simulink model "WholeBody"  (R2023b)
settings: Solver=daessc  StartTime=0.0  StopTime=10  RelTol=1e-3
undefined symbols (not defined in the file): Kd, Ki, Kp, LF, LFstates, LFtrqs, LR, LRstates, LRtrqs, RF, RFstates, RFtrqs, RR, RRstates, RRtrqs, X, Y, Z
libraries: sm_lib x57, nesl_utility x37, SignalEditorBlockLib x1
(part 3 of 3)

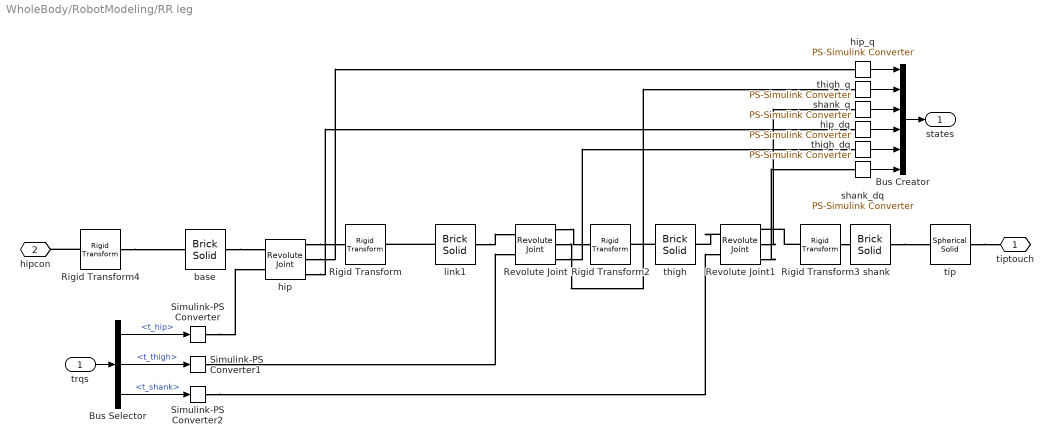
== system WholeBody/RobotModeling/RR leg ==
  trqs : Inport
  Bus Creator : BusCreator  Inputs=6
  Bus Selector : BusSelector  OutputSignals=t_hip,t_thigh,t_shank
  Revolute Joint : sm_lib/Joints/Revolute Joint  JointMode=Normal  SenseConstraintForce=off  SenseConstraintForceX=off  SenseConstraintForceY=off  SenseConstraintForceZ=off  SenseConstraintTorque=off  SenseConstraintTorqueX=off  SenseConstraintTorqueY=off  SenseConstraintTorqueZ=off  SenseTotalForce=off  SenseTotalForceX=off  SenseTotalForceY=off  SenseTotalForceZ=off  SenseTotalTorque=off  SenseTotalTorqueX=off  SenseTotalTorqueY=off  SenseTotalTorqueZ=off  CompositeWrenchDir=FollowerOnBase  CompositeWrenchFrame=BaseFrame  EquilibriumPosition=0  EquilibriumPositionUnits=deg  SpringStiffness=0  SpringStiffnessUnits=N*m/deg  DampingCoefficient=0  DampingCoefficientUnits=N*m/(deg/s)  TorqueActuationMode=InputTorque  MotionActuationMode=ComputedMotion  SensePosition=on  SenseVelocity=on  SenseAcceleration=off  SenseTorqueForce=off  SenseLowerLimitTorqueForce=off  SenseUpperLimitTorqueForce=off  LowerLimitSpecify=off  LowerLimitBound=-90  LowerLimitBoundUnits=deg  LowerLimitStiffness=1e4  LowerLimitStiffnessUnits=N*m/deg  LowerLimitDamping=10  LowerLimitDampingUnits=N*m/(deg/s)  LowerLimitTransitionRegionWidth=0.1  LowerLimitTransitionRegionWidthUnits=deg  UpperLimitSpecify=off  UpperLimitBound=90  UpperLimitBoundUnits=deg  UpperLimitStiffness=1e4  UpperLimitStiffnessUnits=N*m/deg  UpperLimitDamping=10  UpperLimitDampingUnits=N*m/(deg/s)  UpperLimitTransitionRegionWidth=0.1  UpperLimitTransitionRegionWidthUnits=deg  PositionTargetSpecify=off  PositionTargetPriority=High  PositionTargetValue=0  PositionTargetValueUnits=deg  VelocityTargetSpecify=off  VelocityTargetPriority=High  VelocityTargetValue=0  VelocityTargetValueUnits=deg/s
  Revolute Joint1 : sm_lib/Joints/Revolute Joint  JointMode=Normal  SenseConstraintForce=off  SenseConstraintForceX=off  SenseConstraintForceY=off  SenseConstraintForceZ=off  SenseConstraintTorque=off  SenseConstraintTorqueX=off  SenseConstraintTorqueY=off  SenseConstraintTorqueZ=off  SenseTotalForce=off  SenseTotalForceX=off  SenseTotalForceY=off  SenseTotalForceZ=off  SenseTotalTorque=off  SenseTotalTorqueX=off  SenseTotalTorqueY=off  SenseTotalTorqueZ=off  CompositeWrenchDir=FollowerOnBase  CompositeWrenchFrame=BaseFrame  EquilibriumPosition=0  EquilibriumPositionUnits=deg  SpringStiffness=0  SpringStiffnessUnits=N*m/deg  DampingCoefficient=0  DampingCoefficientUnits=N*m/(deg/s)  TorqueActuationMode=InputTorque  MotionActuationMode=ComputedMotion  SensePosition=on  SenseVelocity=on  SenseAcceleration=off  SenseTorqueForce=off  SenseLowerLimitTorqueForce=off  SenseUpperLimitTorqueForce=off  LowerLimitSpecify=off  LowerLimitBound=-90  LowerLimitBoundUnits=deg  LowerLimitStiffness=1e4  LowerLimitStiffnessUnits=N*m/deg  LowerLimitDamping=10  LowerLimitDampingUnits=N*m/(deg/s)  LowerLimitTransitionRegionWidth=0.1  LowerLimitTransitionRegionWidthUnits=deg  UpperLimitSpecify=off  UpperLimitBound=90  UpperLimitBoundUnits=deg  UpperLimitStiffness=1e4  UpperLimitStiffnessUnits=N*m/deg  UpperLimitDamping=10  UpperLimitDampingUnits=N*m/(deg/s)  UpperLimitTransitionRegionWidth=0.1  UpperLimitTransitionRegionWidthUnits=deg  PositionTargetSpecify=off  PositionTargetPriority=High  PositionTargetValue=20  PositionTargetValueUnits=deg  VelocityTargetSpecify=off  VelocityTargetPriority=High  VelocityTargetValue=0  VelocityTargetValueUnits=deg/s
  Rigid Transform : sm_lib/Frames and Transforms/Rigid Transform  TranslationMethod=Cartesian  TranslationStandardOffset=0  TranslationStandardOffsetUnits=m  TranslationStandardAxis=+Z  TranslationCartesianOffset=[0.1 0 0]  TranslationCartesianOffsetUnits=m  TranslationROffset=0  TranslationROffsetUnits=m  TranslationZOffset=0  TranslationZOffsetUnits=m  TranslationThetaOffset=0  TranslationThetaOffsetUnits=deg  RotationMethod=None  RotationAngleUnits=deg  RotationStandardAxis=+Z  RotationAngle=0.0  RotationArbitraryAxis=[0 0 1]  FollAlignAxisA=+X  BaseAlignAxisA=+Y  FollAlignAxisB=+Y  BaseAlignAxisB=+Z  RotationSequenceAxes=FollowerAxes  RotationSequence=XYX  RotationSequenceAngles=[0 0 0]  RotationSequenceAnglesUnits=deg  RotationMatrix=[1 0 0; 0 1 0; 0 0 1]  Quaternion=[1 0 0 0]
  Rigid Transform2 : sm_lib/Frames and Transforms/Rigid Transform  TranslationMethod=Cartesian  TranslationStandardOffset=0  TranslationStandardOffsetUnits=m  TranslationStandardAxis=+Z  TranslationCartesianOffset=[0 -0.4 0]  TranslationCartesianOffsetUnits=m  TranslationROffset=0  TranslationROffsetUnits=m  TranslationZOffset=0  TranslationZOffsetUnits=m  TranslationThetaOffset=0  TranslationThetaOffsetUnits=deg  RotationMethod=None  RotationAngleUnits=deg  RotationStandardAxis=+Z  RotationAngle=0.0  RotationArbitraryAxis=[0 0 1]  FollAlignAxisA=+X  BaseAlignAxisA=+Y  FollAlignAxisB=+Y  BaseAlignAxisB=+Z  RotationSequenceAxes=FollowerAxes  RotationSequence=XYX  RotationSequenceAngles=[0 0 0]  RotationSequenceAnglesUnits=deg  RotationMatrix=[1 0 0; 0 1 0; 0 0 1]  Quaternion=[1 0 0 0]
  Rigid Transform3 : sm_lib/Frames and Transforms/Rigid Transform  TranslationMethod=Cartesian  TranslationStandardOffset=0  TranslationStandardOffsetUnits=m  TranslationStandardAxis=+Z  TranslationCartesianOffset=[0 -0.4 0]  TranslationCartesianOffsetUnits=m  TranslationROffset=0  TranslationROffsetUnits=m  TranslationZOffset=0  TranslationZOffsetUnits=m  TranslationThetaOffset=0  TranslationThetaOffsetUnits=deg  RotationMethod=None  RotationAngleUnits=deg  RotationStandardAxis=+Z  RotationAngle=0.0  RotationArbitraryAxis=[0 0 1]  FollAlignAxisA=+X  BaseAlignAxisA=+Y  FollAlignAxisB=+Y  BaseAlignAxisB=+Z  RotationSequenceAxes=FollowerAxes  RotationSequence=XYX  RotationSequenceAngles=[0 0 0]  RotationSequenceAnglesUnits=deg  RotationMatrix=[1 0 0; 0 1 0; 0 0 1]  Quaternion=[1 0 0 0]
  Rigid Transform4 : sm_lib/Frames and Transforms/Rigid Transform  TranslationMethod=Cartesian  TranslationStandardOffset=0  TranslationStandardOffsetUnits=m  TranslationStandardAxis=+Z  TranslationCartesianOffset=[0.35 0 1.25]  TranslationCartesianOffsetUnits=m  TranslationROffset=0  TranslationROffsetUnits=m  TranslationZOffset=0  TranslationZOffsetUnits=m  TranslationThetaOffset=0  TranslationThetaOffsetUnits=deg  RotationMethod=StandardAxis  RotationAngleUnits=deg  RotationStandardAxis=+Y  RotationAngle=90  RotationArbitraryAxis=[0 0 1]  FollAlignAxisA=+X  BaseAlignAxisA=+Y  FollAlignAxisB=+Y  BaseAlignAxisB=+Z  RotationSequenceAxes=FollowerAxes  RotationSequence=XYX  RotationSequenceAngles=[0 0 0]  RotationSequenceAnglesUnits=deg  RotationMatrix=[1 0 0; 0 1 0; 0 0 1]  Quaternion=[1 0 0 0]
  Simulink-PS Converter : nesl_utility/Simulink-PS Converter  PhysicalDomain=network_engine_domain  SubClassName=ps_input  LeftPortType=input  RightPortType=output  PseudoPeriodic=off  Frequencies=[]  NoiseDistribution=none  NoiseParameters=[]  Unit=1  AffineConversion=off  FilteringAndDerivatives=provide  SimscapeFilterOrder=1  InputFilterTimeConstant=0.001  UdotUserProvided=0
  Simulink-PS Converter1 : nesl_utility/Simulink-PS Converter  PhysicalDomain=network_engine_domain  SubClassName=ps_input  LeftPortType=input  RightPortType=output  PseudoPeriodic=off  Frequencies=[]  NoiseDistribution=none  NoiseParameters=[]  Unit=1  AffineConversion=off  FilteringAndDerivatives=provide  SimscapeFilterOrder=1  InputFilterTimeConstant=0.001  UdotUserProvided=0
  Simulink-PS Converter2 : nesl_utility/Simulink-PS Converter  PhysicalDomain=network_engine_domain  SubClassName=ps_input  LeftPortType=input  RightPortType=output  PseudoPeriodic=off  Frequencies=[]  NoiseDistribution=none  NoiseParameters=[]  Unit=1  AffineConversion=off  FilteringAndDerivatives=provide  SimscapeFilterOrder=1  InputFilterTimeConstant=0.001  UdotUserProvided=0
  base : sm_lib/Body Elements/Brick Solid  GraphicAmbientColor=[0.15 0.15 0.15 1.0]  BasedOnType=Density  BrickDimensions=[0.05 0.05 0.05]  BrickDimensionsUnits=m  CenterOfMass=[0 0 0]  CenterOfMassUnits=m  GraphicDiffuseColor=[0.0 0.8 0.8]  Density=1000  DensityUnits=kg/m^3  DoExposeReferenceFrame=on  GraphicEmissiveColor=[0.0 0.0 0.0 1.0]  ExportEntireGeometry=off  SerializedFrames=<Frames><Frame><Id>Frame1</Id><Value><Name>hip</Name><Origin><Source>GeometricFeature</Source><FeatureName>+z surface</FeatureName></Origin><PrimaryAxis><DefinedDirection>+Z</DefinedDirection><Source>ReferenceFrame</Source><SourceDirection>-X</SourceDirection><FeatureName></FeatureName></PrimaryAxis><SecondaryAxis><DefinedDirection>+X</DefinedDirection><Source>ReferenceFrame</Source><SourceDirection>+Z</SourceDirection><FeatureName></FeatureName></SecondaryAxis></Value></Frame></Frames>  MarkerShape=Sphere  MarkerSize=10  GraphicType=FromGeometry  InertiaType=CalculateFromGeometry  Mass=1  MassUnits=kg  MomentsOfInertia=[1 1 1]  MomentsOfInertiaUnits=kg*m^2  GraphicOpacity=1.0  ProductsOfInertia=[0 0 0]  ProductsOfInertiaUnits=kg*m^2  GraphicShininess=75  GraphicSpecularColor=[0.5 0.5 0.5 1.0]  GraphicVisPropType=SimpleVisualProperties
  hip : sm_lib/Joints/Revolute Joint  JointMode=Normal  SenseConstraintForce=off  SenseConstraintForceX=off  SenseConstraintForceY=off  SenseConstraintForceZ=off  SenseConstraintTorque=off  SenseConstraintTorqueX=off  SenseConstraintTorqueY=off  SenseConstraintTorqueZ=off  SenseTotalForce=off  SenseTotalForceX=off  SenseTotalForceY=off  SenseTotalForceZ=off  SenseTotalTorque=off  SenseTotalTorqueX=off  SenseTotalTorqueY=off  SenseTotalTorqueZ=off  CompositeWrenchDir=FollowerOnBase  CompositeWrenchFrame=BaseFrame  EquilibriumPosition=0  EquilibriumPositionUnits=deg  SpringStiffness=0  SpringStiffnessUnits=N*m/deg  DampingCoefficient=0  DampingCoefficientUnits=N*m/(deg/s)  TorqueActuationMode=InputTorque  MotionActuationMode=ComputedMotion  SensePosition=on  SenseVelocity=on  SenseAcceleration=off  SenseTorqueForce=off  SenseLowerLimitTorqueForce=off  SenseUpperLimitTorqueForce=off  LowerLimitSpecify=off  LowerLimitBound=-90  LowerLimitBoundUnits=deg  LowerLimitStiffness=1e4  LowerLimitStiffnessUnits=N*m/deg  LowerLimitDamping=10  LowerLimitDampingUnits=N*m/(deg/s)  LowerLimitTransitionRegionWidth=0.1  LowerLimitTransitionRegionWidthUnits=deg  UpperLimitSpecify=off  UpperLimitBound=90  UpperLimitBoundUnits=deg  UpperLimitStiffness=1e4  UpperLimitStiffnessUnits=N*m/deg  UpperLimitDamping=10  UpperLimitDampingUnits=N*m/(deg/s)  UpperLimitTransitionRegionWidth=0.1  UpperLimitTransitionRegionWidthUnits=deg  PositionTargetSpecify=off  PositionTargetPriority=High  PositionTargetValue=0  PositionTargetValueUnits=deg  VelocityTargetSpecify=off  VelocityTargetPriority=High  VelocityTargetValue=0  VelocityTargetValueUnits=deg/s
  hip_dq : nesl_utility/PS-Simulink Converter  PhysicalDomain=network_engine_domain  SubClassName=ps_output  LeftPortType=input  RightPortType=output  PseudoPeriodic=off  Frequencies=[]  VectorFormat=inherit  Unit=inherit  AffineConversion=off
  hip_q : nesl_utility/PS-Simulink Converter  PhysicalDomain=network_engine_domain  SubClassName=ps_output  LeftPortType=input  RightPortType=output  PseudoPeriodic=off  Frequencies=[]  VectorFormat=inherit  Unit=inherit  AffineConversion=off
  link1 : sm_lib/Body Elements/Brick Solid  GraphicAmbientColor=[0.15 0.15 0.15 1.0]  BasedOnType=Mass  BrickDimensions=[0.2 0.05 0.05]  BrickDimensionsUnits=m  CenterOfMass=[0 0 0]  CenterOfMassUnits=m  GraphicDiffuseColor=[0.5 0.5 0.5]  Density=1000  DensityUnits=kg/m^3  DoExposeReferenceFrame=on  GraphicEmissiveColor=[0.0 0.0 0.0 1.0]  ExportEntireGeometry=off  SerializedFrames=<Frames><Frame><Id>Frame1</Id><Value><Name>thigh</Name><Origin><Source>GeometricFeature</Source><FeatureName>+x surface</FeatureName></Origin><PrimaryAxis><DefinedDirection>+Z</DefinedDirection><Source>ReferenceFrame</Source><SourceDirection>+X</SourceDirection><FeatureName></FeatureName></PrimaryAxis><SecondaryAxis><DefinedDirection>+X</DefinedDirection><Source>ReferenceFrame</Source><SourceDirection>-Z</SourceDirection><FeatureName></FeatureName></SecondaryAxis></Value></Frame></Frames>  MarkerShape=Sphere  MarkerSize=10  GraphicType=FromGeometry  InertiaType=CalculateFromGeometry  Mass=0.2  MassUnits=kg  MomentsOfInertia=[1 1 1]  MomentsOfInertiaUnits=kg*m^2  GraphicOpacity=1.0  ProductsOfInertia=[0 0 0]  ProductsOfInertiaUnits=kg*m^2  GraphicShininess=75  GraphicSpecularColor=[0.5 0.5 0.5 1.0]  GraphicVisPropType=SimpleVisualProperties
  shank : sm_lib/Body Elements/Brick Solid  GraphicAmbientColor=[0.15 0.15 0.15 1.0]  BasedOnType=Mass  BrickDimensions=[0.07 0.8 0.07]  BrickDimensionsUnits=m  CenterOfMass=[0 0 0]  CenterOfMassUnits=m  GraphicDiffuseColor=[0.5 0.5 0.5]  Density=1000  DensityUnits=kg/m^3  DoExposeReferenceFrame=on  GraphicEmissiveColor=[0.0 0.0 0.0 1.0]  ExportEntireGeometry=off  SerializedFrames=<Frames><Frame><Id>Frame1</Id><Value><Name>F1</Name><Origin><Source>GeometricFeature</Source><FeatureName>-y surface</FeatureName></Origin><PrimaryAxis><DefinedDirection>+Z</DefinedDirection><Source>ReferenceFrame</Source><SourceDirection>+Z</SourceDirection><FeatureName></FeatureName></PrimaryAxis><SecondaryAxis><DefinedDirection>+X</DefinedDirection><Source>ReferenceFrame</Source><SourceDirection>+X</SourceDirection><FeatureName></FeatureName></SecondaryAxis></Value></Frame></Frames>  MarkerShape=Sphere  MarkerSize=10  GraphicType=FromGeometry  InertiaType=CalculateFromGeometry  Mass=0.5  MassUnits=kg  MomentsOfInertia=[1 1 1]  MomentsOfInertiaUnits=kg*m^2  GraphicOpacity=1.0  ProductsOfInertia=[0 0 0]  ProductsOfInertiaUnits=kg*m^2  GraphicShininess=75  GraphicSpecularColor=[0.5 0.5 0.5 1.0]  GraphicVisPropType=SimpleVisualProperties
  shank_dq : nesl_utility/PS-Simulink Converter  PhysicalDomain=network_engine_domain  SubClassName=ps_output  LeftPortType=input  RightPortType=output  PseudoPeriodic=off  Frequencies=[]  VectorFormat=inherit  Unit=inherit  AffineConversion=off
  shank_q : nesl_utility/PS-Simulink Converter  PhysicalDomain=network_engine_domain  SubClassName=ps_output  LeftPortType=input  RightPortType=output  PseudoPeriodic=off  Frequencies=[]  VectorFormat=inherit  Unit=inherit  AffineConversion=off
  thigh : sm_lib/Body Elements/Brick Solid  GraphicAmbientColor=[0.15 0.15 0.15 1.0]  BasedOnType=Mass  BrickDimensions=[0.07 0.8 0.07]  BrickDimensionsUnits=m  CenterOfMass=[0 0 0]  CenterOfMassUnits=m  GraphicDiffuseColor=[0.5 0.5 0.5]  Density=1000  DensityUnits=kg/m^3  DoExposeReferenceFrame=on  GraphicEmissiveColor=[0.0 0.0 0.0 1.0]  ExportEntireGeometry=off  SerializedFrames=<Frames><Frame><Id>Frame1</Id><Value><Name>F1</Name><Origin><Source>GeometricFeature</Source><FeatureName>-y surface</FeatureName></Origin><PrimaryAxis><DefinedDirection>+Z</DefinedDirection><Source>ReferenceFrame</Source><SourceDirection>+Z</SourceDirection><FeatureName></FeatureName></PrimaryAxis><SecondaryAxis><DefinedDirection>+Y</DefinedDirection><Source>ReferenceFrame</Source><SourceDirection>+Y</SourceDirection><FeatureName></FeatureName></SecondaryAxis></Value></Frame></Frames>  MarkerShape=Sphere  MarkerSize=10  GraphicType=FromGeometry  InertiaType=CalculateFromGeometry  Mass=0.5  MassUnits=kg  MomentsOfInertia=[1 1 1]  MomentsOfInertiaUnits=kg*m^2  GraphicOpacity=1.0  ProductsOfInertia=[0 0 0]  ProductsOfInertiaUnits=kg*m^2  GraphicShininess=75  GraphicSpecularColor=[0.5 0.5 0.5 1.0]  GraphicVisPropType=SimpleVisualProperties
  thigh_dq : nesl_utility/PS-Simulink Converter  PhysicalDomain=network_engine_domain  SubClassName=ps_output  LeftPortType=input  RightPortType=output  PseudoPeriodic=off  Frequencies=[]  VectorFormat=inherit  Unit=inherit  AffineConversion=off
  thigh_q : nesl_utility/PS-Simulink Converter  PhysicalDomain=network_engine_domain  SubClassName=ps_output  LeftPortType=input  RightPortType=output  PseudoPeriodic=off  Frequencies=[]  VectorFormat=inherit  Unit=inherit  AffineConversion=off
  tip : sm_lib/Body Elements/Spherical Solid  GraphicAmbientColor=[0.15 0.15 0.15 1.0]  BasedOnType=Mass  CenterOfMass=[0 0 0]  CenterOfMassUnits=m  GraphicDiffuseColor=[0.0 1.0 0.6]  Density=1000  DensityUnits=kg/m^3  DoExposeReferenceFrame=on  GraphicEmissiveColor=[0.0 0.0 0.0 1.0]  ExportEntireGeometry=on  SerializedExposedGeometries=<exposedGeometries><exposedGeom><rawGeomId>entire</rawGeomId><exposedGeomId>G</exposedGeomId></exposedGeom></exposedGeometries>  SerializedFrames=<Frames/>  MarkerShape=Sphere  MarkerSize=10  GraphicType=FromGeometry  InertiaType=CalculateFromGeometry  Mass=0.01  MassUnits=kg  MomentsOfInertia=[1 1 1]  MomentsOfInertiaUnits=kg*m^2  GraphicOpacity=1.0  ProductsOfInertia=[0 0 0]  ProductsOfInertiaUnits=kg*m^2  GraphicShininess=75  GraphicSpecularColor=[0.5 0.5 0.5 1.0]  SphereRadius=0.08  SphereRadiusUnits=m  GraphicVisPropType=SimpleVisualProperties
  tiptouch : PMIOPort  Side=Left
  hipcon : PMIOPort  Port=2  Side=Left
  states : Outport
  wires:
  Bus Creator/1 -> states/1
  Bus Selector/2 -> Simulink-PS Converter1/1  "<t_thigh>"
  thigh_q/1 -> Bus Creator/2
  thigh_dq/1 -> Bus Creator/5
  hip_q/1 -> Bus Creator/1
  Bus Selector/1 -> Simulink-PS Converter/1  "<t_hip>"
  hip_dq/1 -> Bus Creator/4
  Bus Selector/3 -> Simulink-PS Converter2/1  "<t_shank>"
  shank_dq/1 -> Bus Creator/6
  shank_q/1 -> Bus Creator/3
  trqs/1 -> Bus Selector/1
  connections:
  tip/LConn1 -- tiptouch/RConn1
  Revolute Joint1/RConn3 -- shank_dq/LConn1
  Revolute Joint1/RConn2 -- shank_q/LConn1
  Simulink-PS Converter2/RConn1 -- Revolute Joint1/LConn2
  Revolute Joint/RConn2 -- thigh_q/LConn1
  Simulink-PS Converter/RConn1 -- hip/LConn2
  hip/RConn3 -- hip_dq/LConn1
  base/LConn1 -- hip/LConn1
  hip/RConn1 -- Rigid Transform/LConn1
  Simulink-PS Converter1/RConn1 -- Revolute Joint/LConn2
  hip/RConn2 -- hip_q/LConn1
  link1/RConn1 -- Rigid Transform/RConn1
  Revolute Joint1/LConn1 -- thigh/LConn1
  Rigid Transform3/LConn1 -- Revolute Joint1/RConn1
  thigh/RConn1 -- Rigid Transform2/RConn1
  Rigid Transform3/RConn1 -- shank/RConn1
  Revolute Joint/RConn3 -- thigh_dq/LConn1
  Revolute Joint/RConn1 -- Rigid Transform2/LConn1
  Rigid Transform4/LConn1 -- hipcon/RConn1
  shank/LConn1 -- tip/RConn1
  Rigid Transform4/RConn1 -- base/RConn1
  link1/LConn1 -- Revolute Joint/LConn1

== matlab function WholeBody/Behavior/RR ==
  data: pos input; qs output; legStrucs input
function qs = Leg3DiKinematic(pos,legStrucs)
% coder. extrinsic('InvKine');
% qs = [0;0;0];
% qs = InvKine(pos,legStrucs);

x = pos(3);
y = pos(2);
z = pos(1);
l1 = legStrucs(1);
l2 = legStrucs(2);
l3 = legStrucs(3);

L = sqrt(x^2 + y^2 - l1^2);

t1 = atan2((y * l1 + x * L),(x * l1 - y * L))

% 求解 th3
t3 = pi - acos((l2^2 + l3^2 - (x^2 + y^2 + z^2 - l1^2))/(2*l2*l3));

t2_t = -(z + (l3*(y - (l1*(imag(l1*x) + real(l1*y) - imag(y*(- l1^2 + x^2 + y^2)^(1/2)) + real(x*(- l1^2 + x^2 + y^2)^(1/2))))/abs(l1*x - y*(- l1^2 + x^2 + y^2)^(1/2) + l1*y*1i + x*(- l1^2 + x^2 + y^2)^(1/2)*1i))*(1 - (l1^2 + l2^2 + l3^2 - x^2 - y^2 - z^2)^2/(4*l2^2*l3^2))^(1/2))/((l2*(imag(l1*y) - real(l1*x) + imag(x*(- l1^2 + x^2 + y^2)^(1/2)) + real(y*(- l1^2 + x^2 + y^2)^(1/2))))/abs(l1*x - y*(- l1^2 + x^2 + y^2)^(1/2) + l1*y*1i + x*(- l1^2 + x^2 + y^2)^(1/2)*1i) - ((imag(l1*y) - real(l1*x) + imag(x*(- l1^2 + x^2 + y^2)^(1/2)) + real(y*(- l1^2 + x^2 + y^2)^(1/2)))*(l1^2 + l2^2 + l3^2 - x^2 - y^2 - z^2))/(2*l2*abs(l1*x - y*(- l1^2 + x^2 + y^2)^(1/2) + l1*y*1i + x*(- l1^2 + x^2 + y^2)^(1/2)*1i))))/(l2 - l3*((l1^2 + l2^2 + l3^2 - x^2 - y^2 - z^2)/(2*l2*l3) + (l3*((l1^2 + l2^2 + l3^2 - x^2 - y^2 - z^2)^2/(4*l2^2*l3^2) - 1)*(imag(l1*y) - real(l1*x) + imag(x*(- l1^2 + x^2 + y^2)^(1/2)) + real(y*(- l1^2 + x^2 + y^2)^(1/2))))/(abs(l1*x - y*(- l1^2 + x^2 + y^2)^(1/2) + l1*y*1i + x*(- l1^2 + x^2 + y^2)^(1/2)*1i)*((l2*(imag(l1*y) - real(l1*x) + imag(x*(- l1^2 + x^2 + y^2)^(1/2)) + real(y*(- l1^2 + x^2 + y^2)^(1/2))))/abs(l1*x - y*(- l1^2 + x^2 + y^2)^(1/2) + l1*y*1i + x*(- l1^2 + x^2 + y^2)^(1/2)*1i) - ((imag(l1*y) - real(l1*x) + imag(x*(- l1^2 + x^2 + y^2)^(1/2)) + real(y*(- l1^2 + x^2 + y^2)^(1/2)))*(l1^2 + l2^2 + l3^2 - x^2 - y^2 - z^2))/(2*l2*abs(l1*x - y*(- l1^2 + x^2 + y^2)^(1/2) + l1*y*1i + x*(- l1^2 + x^2 + y^2)^(1/2)*1i))))));

t2 = asin(t2_t);

qs = [t1;t2;t3];

== matlab function WholeBody/Behavior/RF ==
  data: pos input; qs output; legStrucs input
function qs = Leg3DiKinematic(pos,legStrucs)
x = pos(3);
y = pos(2);
z = pos(1);
l1 = legStrucs(1);
l2 = legStrucs(2);
l3 = legStrucs(3);

L = sqrt(x^2 + y^2 - l1^2);

t1 = atan2((y * l1 + x * L),(x * l1 - y * L));

% 求解 th3
t3 = pi - acos((l2^2 + l3^2 - (x^2 + y^2 + z^2 - l1^2))/(2*l2*l3));

t2_t = -(z + (l3*(y - (l1*(imag(l1*x) + real(l1*y) - imag(y*(- l1^2 + x^2 + y^2)^(1/2)) + real(x*(- l1^2 + x^2 + y^2)^(1/2))))/abs(l1*x - y*(- l1^2 + x^2 + y^2)^(1/2) + l1*y*1i + x*(- l1^2 + x^2 + y^2)^(1/2)*1i))*(1 - (l1^2 + l2^2 + l3^2 - x^2 - y^2 - z^2)^2/(4*l2^2*l3^2))^(1/2))/((l2*(imag(l1*y) - real(l1*x) + imag(x*(- l1^2 + x^2 + y^2)^(1/2)) + real(y*(- l1^2 + x^2 + y^2)^(1/2))))/abs(l1*x - y*(- l1^2 + x^2 + y^2)^(1/2) + l1*y*1i + x*(- l1^2 + x^2 + y^2)^(1/2)*1i) - ((imag(l1*y) - real(l1*x) + imag(x*(- l1^2 + x^2 + y^2)^(1/2)) + real(y*(- l1^2 + x^2 + y^2)^(1/2)))*(l1^2 + l2^2 + l3^2 - x^2 - y^2 - z^2))/(2*l2*abs(l1*x - y*(- l1^2 + x^2 + y^2)^(1/2) + l1*y*1i + x*(- l1^2 + x^2 + y^2)^(1/2)*1i))))/(l2 - l3*((l1^2 + l2^2 + l3^2 - x^2 - y^2 - z^2)/(2*l2*l3) + (l3*((l1^2 + l2^2 + l3^2 - x^2 - y^2 - z^2)^2/(4*l2^2*l3^2) - 1)*(imag(l1*y) - real(l1*x) + imag(x*(- l1^2 + x^2 + y^2)^(1/2)) + real(y*(- l1^2 + x^2 + y^2)^(1/2))))/(abs(l1*x - y*(- l1^2 + x^2 + y^2)^(1/2) + l1*y*1i + x*(- l1^2 + x^2 + y^2)^(1/2)*1i)*((l2*(imag(l1*y) - real(l1*x) + imag(x*(- l1^2 + x^2 + y^2)^(1/2)) + real(y*(- l1^2 + x^2 + y^2)^(1/2))))/abs(l1*x - y*(- l1^2 + x^2 + y^2)^(1/2) + l1*y*1i + x*(- l1^2 + x^2 + y^2)^(1/2)*1i) - ((imag(l1*y) - real(l1*x) + imag(x*(- l1^2 + x^2 + y^2)^(1/2)) + real(y*(- l1^2 + x^2 + y^2)^(1/2)))*(l1^2 + l2^2 + l3^2 - x^2 - y^2 - z^2))/(2*l2*abs(l1*x - y*(- l1^2 + x^2 + y^2)^(1/2) + l1*y*1i + x*(- l1^2 + x^2 + y^2)^(1/2)*1i))))));

t2 = asin(t2_t);

qs = [t1;t2;t3];

== matlab function WholeBody/Behavior/LR ==
  data: pos input; qs output; legStrucs input
function qs = Leg3DiKinematic(pos,legStrucs)
% coder. extrinsic('InvKine');
% qs = [0;0;0];
% qs = InvKine(pos,legStrucs);

x = pos(3);
y = pos(2);
z = pos(1);
l1 = legStrucs(1);
l2 = legStrucs(2);
l3 = legStrucs(3);

L = sqrt(x^2 + y^2 - l1^2);

t1 = atan2((y * l1 + x * L),(x * l1 - y * L));

% 求解 th3
t3 = pi - acos((l2^2 + l3^2 - (x^2 + y^2 + z^2 - l1^2))/(2*l2*l3));

t2_t = -(z + (l3*(y - (l1*(imag(l1*x) + real(l1*y) - imag(y*(- l1^2 + x^2 + y^2)^(1/2)) + real(x*(- l1^2 + x^2 + y^2)^(1/2))))/abs(l1*x - y*(- l1^2 + x^2 + y^2)^(1/2) + l1*y*1i + x*(- l1^2 + x^2 + y^2)^(1/2)*1i))*(1 - (l1^2 + l2^2 + l3^2 - x^2 - y^2 - z^2)^2/(4*l2^2*l3^2))^(1/2))/((l2*(imag(l1*y) - real(l1*x) + imag(x*(- l1^2 + x^2 + y^2)^(1/2)) + real(y*(- l1^2 + x^2 + y^2)^(1/2))))/abs(l1*x - y*(- l1^2 + x^2 + y^2)^(1/2) + l1*y*1i + x*(- l1^2 + x^2 + y^2)^(1/2)*1i) - ((imag(l1*y) - real(l1*x) + imag(x*(- l1^2 + x^2 + y^2)^(1/2)) + real(y*(- l1^2 + x^2 + y^2)^(1/2)))*(l1^2 + l2^2 + l3^2 - x^2 - y^2 - z^2))/(2*l2*abs(l1*x - y*(- l1^2 + x^2 + y^2)^(1/2) + l1*y*1i + x*(- l1^2 + x^2 + y^2)^(1/2)*1i))))/(l2 - l3*((l1^2 + l2^2 + l3^2 - x^2 - y^2 - z^2)/(2*l2*l3) + (l3*((l1^2 + l2^2 + l3^2 - x^2 - y^2 - z^2)^2/(4*l2^2*l3^2) - 1)*(imag(l1*y) - real(l1*x) + imag(x*(- l1^2 + x^2 + y^2)^(1/2)) + real(y*(- l1^2 + x^2 + y^2)^(1/2))))/(abs(l1*x - y*(- l1^2 + x^2 + y^2)^(1/2) + l1*y*1i + x*(- l1^2 + x^2 + y^2)^(1/2)*1i)*((l2*(imag(l1*y) - real(l1*x) + imag(x*(- l1^2 + x^2 + y^2)^(1/2)) + real(y*(- l1^2 + x^2 + y^2)^(1/2))))/abs(l1*x - y*(- l1^2 + x^2 + y^2)^(1/2) + l1*y*1i + x*(- l1^2 + x^2 + y^2)^(1/2)*1i) - ((imag(l1*y) - real(l1*x) + imag(x*(- l1^2 + x^2 + y^2)^(1/2)) + real(y*(- l1^2 + x^2 + y^2)^(1/2)))*(l1^2 + l2^2 + l3^2 - x^2 - y^2 - z^2))/(2*l2*abs(l1*x - y*(- l1^2 + x^2 + y^2)^(1/2) + l1*y*1i + x*(- l1^2 + x^2 + y^2)^(1/2)*1i))))));

t2 = asin(t2_t);

qs = [t1;t2;t3];

== matlab function WholeBody/Behavior/LF ==
  data: pos input; qs output; legStrucs input
function qs = Leg3DiKinematic(pos,legStrucs)
% coder. extrinsic('InvKine');
% qs = [0;0;0];
% qs = InvKine(pos,legStrucs);

x = pos(3);
y = pos(2);
z = pos(1);
l1 = legStrucs(1);
l2 = legStrucs(2);
l3 = legStrucs(3);

L = sqrt(x^2 + y^2 - l1^2);

t1 = atan2((y * l1 + x * L),(x * l1 - y * L));

% 求解 th3
t3 = pi - acos((l2^2 + l3^2 - (x^2 + y^2 + z^2 - l1^2))/(2*l2*l3));

t2_t = -(z + (l3*(y - (l1*(imag(l1*x) + real(l1*y) - imag(y*(- l1^2 + x^2 + y^2)^(1/2)) + real(x*(- l1^2 + x^2 + y^2)^(1/2))))/abs(l1*x - y*(- l1^2 + x^2 + y^2)^(1/2) + l1*y*1i + x*(- l1^2 + x^2 + y^2)^(1/2)*1i))*(1 - (l1^2 + l2^2 + l3^2 - x^2 - y^2 - z^2)^2/(4*l2^2*l3^2))^(1/2))/((l2*(imag(l1*y) - real(l1*x) + imag(x*(- l1^2 + x^2 + y^2)^(1/2)) + real(y*(- l1^2 + x^2 + y^2)^(1/2))))/abs(l1*x - y*(- l1^2 + x^2 + y^2)^(1/2) + l1*y*1i + x*(- l1^2 + x^2 + y^2)^(1/2)*1i) - ((imag(l1*y) - real(l1*x) + imag(x*(- l1^2 + x^2 + y^2)^(1/2)) + real(y*(- l1^2 + x^2 + y^2)^(1/2)))*(l1^2 + l2^2 + l3^2 - x^2 - y^2 - z^2))/(2*l2*abs(l1*x - y*(- l1^2 + x^2 + y^2)^(1/2) + l1*y*1i + x*(- l1^2 + x^2 + y^2)^(1/2)*1i))))/(l2 - l3*((l1^2 + l2^2 + l3^2 - x^2 - y^2 - z^2)/(2*l2*l3) + (l3*((l1^2 + l2^2 + l3^2 - x^2 - y^2 - z^2)^2/(4*l2^2*l3^2) - 1)*(imag(l1*y) - real(l1*x) + imag(x*(- l1^2 + x^2 + y^2)^(1/2)) + real(y*(- l1^2 + x^2 + y^2)^(1/2))))/(abs(l1*x - y*(- l1^2 + x^2 + y^2)^(1/2) + l1*y*1i + x*(- l1^2 + x^2 + y^2)^(1/2)*1i)*((l2*(imag(l1*y) - real(l1*x) + imag(x*(- l1^2 + x^2 + y^2)^(1/2)) + real(y*(- l1^2 + x^2 + y^2)^(1/2))))/abs(l1*x - y*(- l1^2 + x^2 + y^2)^(1/2) + l1*y*1i + x*(- l1^2 + x^2 + y^2)^(1/2)*1i) - ((imag(l1*y) - real(l1*x) + imag(x*(- l1^2 + x^2 + y^2)^(1/2)) + real(y*(- l1^2 + x^2 + y^2)^(1/2)))*(l1^2 + l2^2 + l3^2 - x^2 - y^2 - z^2))/(2*l2*abs(l1*x - y*(- l1^2 + x^2 + y^2)^(1/2) + l1*y*1i + x*(- l1^2 + x^2 + y^2)^(1/2)*1i))))));

t2 = asin(t2_t);

qs = [t1;t2;t3];

== matlab function WholeBody/Behavior/MATLAB Function ==
  data: pos input; plRR output; att input; plRF output; plLR output; plLF output
function [plRR,plRF,plLR,plLF]= BodyKine(pos,att)
x = pos(1);
y = pos(2);
z = pos(3);
alpha = att(1);
beta = att(2);
gamma = att(3);

%% 因为不希望足端发生滑移，所以我们有已经固定的各个 p_{si}
psRR = [0;0;0;1];
psRF = [2.5;0;0;1];
psLR = [0;0;-0.7;1];
psLF = [2.5;0;-0.7;1];

%% 根据我们希望的机体目标状态，我们可以求解出世界坐标系到机体坐标系的齐次变换矩阵
% 得出绕各个轴的旋转矩阵
Rz = [cos(alpha) -sin(alpha) 0;
      sin(alpha) cos(alpha) 0;
      0 0 1];
Ry = [cos(beta) 0 sin(beta);
      0 1 0;
      -sin(beta) 0 cos(beta)];
Rx = [1 0 0;
      0 cos(gamma) -sin(gamma);
      0 sin(gamma) cos(gamma)];
% 得出机体坐标系原点在世界坐标系中的坐标
pbRR0 = [-1.25;-1;0.35+0.2];
pd = [x;y;z];

Tbs = [(Rz*Ry*Rx)' -(Rz*Ry*Rx)'*(-pbRR0+pd);
        zeros(1,3) ones(1,1)];

%% 根据齐次变换矩阵，我们可以求解机体坐标系下的足端位置
pbRR = Tbs * psRR;
pbRF = Tbs * psRF;
pbLR = Tbs * psLR;
pbLF = Tbs * psLF;

%% 再求出单腿坐标系下的足端位置，用单腿逆运动学得到各个关节角度就可以了
plRR = pbRR(1:3,:) - [-1.25;0;0.35];
plRF = pbRF(1:3,:) - [1.25;0;0.35];
plLR = pbLR(1:3,:) - [-1.25;0;-0.35];
plLF = pbLF(1:3,:) - [1.25;0;-0.35];

== matlab function WholeBody/LegController/RR controller/MATLAB Function1 ==
  data: t_hip output; t_thigh output; t_shank output; q1 input; q2 input; q3 input; dq1 input; dq2 input; dq3 input; ei input size=[3 1]; ei output size=[3 1]; kp input; ki input; kd input; q_des input
function [t_hip,t_thigh,t_shank,ei] = leg_controller(q1,q2,q3,dq1,dq2,dq3,ei,kp,ki,kd,q_des)
isRight = 1;

q_states = [q1;q2;q3];
dq_states = [dq1;dq2;dq3];
q_des = isRight * q_des;
dq_des = [0;0;0];

e_q = q_des - q_states;
e_dq = dq_des - dq_states;

%PID参数
tqs = kp .* e_q + kd' .* e_dq + ki .* ei; %系统PID控制器输出序列

t_hip = tqs(1);
t_thigh = tqs(2);
t_shank = tqs(3);
ei = ei + e_q;
end

== matlab function WholeBody/LegController/RF controller1/MATLAB Function1 ==
  data: t_hip output; t_thigh output; t_shank output; q1 input; q2 input; q3 input; dq1 input; dq2 input; dq3 input; ei input size=[3 1]; ei output size=[3 1]; kp input; ki input; kd input; q_des input
function [t_hip,t_thigh,t_shank,ei] = leg_controller(q1,q2,q3,dq1,dq2,dq3,ei,kp,ki,kd,q_des)
isRight = 1;

q_states = [q1;q2;q3];
dq_states = [dq1;dq2;dq3];
q_des = isRight * q_des;
dq_des = [0;0;0];

e_q = q_des - q_states;
e_dq = dq_des - dq_states;

%PID参数
tqs = kp .* e_q + kd' .* e_dq + ki .* ei; %系统PID控制器输出序列

t_hip = tqs(1);
t_thigh = tqs(2);
t_shank = tqs(3);
ei = ei + e_q;
end

== matlab function WholeBody/LegController/LR controller2/MATLAB Function1 ==
  data: t_hip output; t_thigh output; t_shank output; q1 input; q2 input; q3 input; dq1 input; dq2 input; dq3 input; ei input size=[3 1]; ei output size=[3 1]; kp input; ki input; kd input; q_des input
function [t_hip,t_thigh,t_shank,ei] = leg_controller(q1,q2,q3,dq1,dq2,dq3,ei,kp,ki,kd,q_des)
isRight = -1;

q_states = [q1;q2;q3];
dq_states = [dq1;dq2;dq3];
q_des = isRight * q_des;
dq_des = [0;0;0];

e_q = q_des - q_states;
e_dq = dq_des - dq_states;

%PID参数
tqs = kp .* e_q + kd' .* e_dq + ki .* ei; %系统PID控制器输出序列

t_hip = tqs(1);
t_thigh = tqs(2);
t_shank = tqs(3);
ei = ei + e_q;
end

== matlab function WholeBody/LegController/LF controller3/MATLAB Function1 ==
  data: t_hip output; t_thigh output; t_shank output; q1 input; q2 input; q3 input; dq1 input; dq2 input; dq3 input; ei input size=[3 1]; ei output size=[3 1]; kp input; ki input; kd input; q_des input
function [t_hip,t_thigh,t_shank,ei] = leg_controller(q1,q2,q3,dq1,dq2,dq3,ei,kp,ki,kd,q_des)
isRight = -1;

q_states = [q1;q2;q3];
dq_states = [dq1;dq2;dq3];
q_des = isRight * q_des;
dq_des = [0;0;0];

e_q = q_des - q_states;
e_dq = dq_des - dq_states;

%PID参数
tqs = kp .* e_q + kd' .* e_dq + ki .* ei; %系统PID控制器输出序列

t_hip = tqs(1);
t_thigh = tqs(2);
t_shank = tqs(3);
ei = ei + e_q;
end
